simulink model "SmoothModel"  (R2020a)
settings: Solver=FixedStepAuto  StartTime=0  StopTime=10.67  FixedStep=0.01  RelTol=1e-3
undefined symbols (not defined in the file): delay, PSM, VSM
settings Model: Creator=Brock  LastModifiedBy=Brock

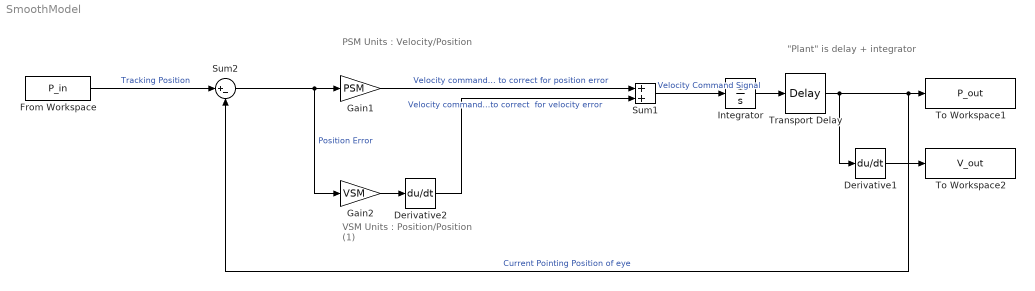
== system SmoothModel ==
  note: "Plant" is delay + integrator
  note: PSM Units : Velocity/Position
  note: VSM Units : Position/Position (1)
  Derivative1 : Derivative
  Derivative2 : Derivative
  From Workspace : FromWorkspace  VariableName=P_in
  Gain1 : Gain  Gain=PSM
  Gain2 : Gain  Gain=VSM
  Integrator : Integrator
  Sum1 : Sum
  Sum2 : Sum  Inputs=|+-
  To Workspace1 : ToWorkspace  VariableName=P_out  SampleTime=-1
  To Workspace2 : ToWorkspace  VariableName=V_out  SampleTime=-1
  Transport Delay : TransportDelay  DelayTime=delay
  wires:
  Sum2/1 -> Gain1/1, Gain2/1  "Position Error"
  Gain1/1 -> Sum1/1  "Velocity command to correct for position error"
  Transport Delay/1 -> Derivative1/1, To Workspace1/1, Sum2/2  "Current Pointing Position of eye"
  Sum1/1 -> Integrator/1  "Velocity Command Signal"
  Derivative2/1 -> Sum1/2  "Velocity command to correct  for velocity error"
  From Workspace/1 -> Sum2/1  "Tracking Position"
  Gain2/1 -> Derivative2/1
  Integrator/1 -> Transport Delay/1
  Derivative1/1 -> To Workspace2/1
